simulink model "Regen"  (R2023b)
settings: Solver=VariableStepAuto  StartTime=0.0  StopTime=800.0  RelTol=1e-3
libraries: simulink x1
settings Model: Creator=joser  LastModifiedBy=joser

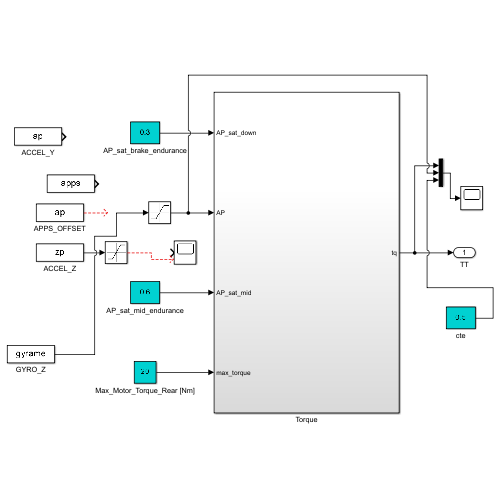
[thumbnail: Simulink's stored preview of the top-level diagram]
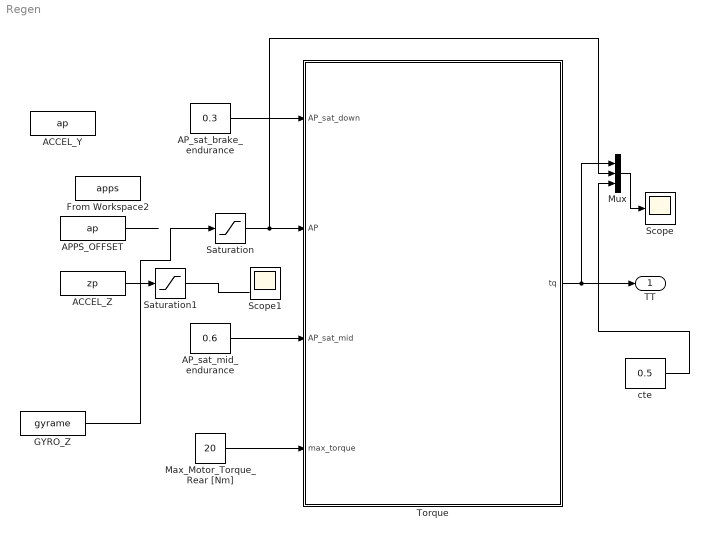
== system Regen ==
  ACCEL_Y : FromWorkspace  VariableName=ap  SampleTime=0.005
  ACCEL_Z : FromWorkspace  VariableName=zp  SampleTime=0.005
  APPS_OFFSET : FromWorkspace  VariableName=ap  SampleTime=0.005
  AP_sat_brake_endurance : Constant  Value=0.3
  AP_sat_mid_endurance : Constant  Value=0.6
  From Workspace2 : FromWorkspace  VariableName=apps  SampleTime=0.005
  GYRO_Z : FromWorkspace  VariableName=gyrame  SampleTime=0.005
  Max_Motor_Torque_Rear [Nm] : Constant  Value=20
  Mux : Mux  Inputs=3
  Saturation : Saturate  UpperLimit=1  LowerLimit=0
  Saturation1 : Saturate  UpperLimit=1  LowerLimit=0
  Scope : Scope
  Scope1 : Scope
  Torque : Subsystem
  cte : Constant  Value=0.5
  TT : Outport
  wires:
  Torque/1(tq) -> Mux/1, TT/1
  AP_sat_brake_endurance/1 -> Torque/1(AP_sat_down)
  Max_Motor_Torque_Rear [Nm]/1 -> Torque/4(max_torque)
  APPS_OFFSET/1 -> ?
  AP_sat_mid_endurance/1 -> Torque/3(AP_sat_mid)
  ACCEL_Z/1 -> Saturation1/1
  Saturation1/1 -> ?
  Mux/1 -> Scope/1
  Saturation/1 -> Mux/2, Torque/2(AP)
  cte/1 -> Mux/3
  GYRO_Z/1 -> Saturation/1

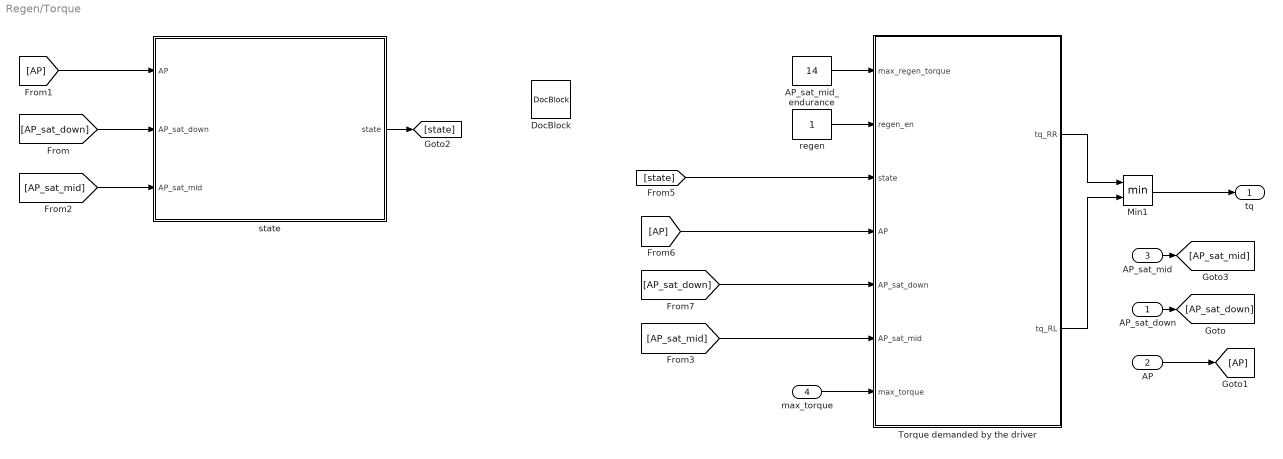
== system Regen/Torque ==
  AP_sat_down : Inport
  AP : Inport  Port=2
  AP_sat_mid : Inport  Port=3
  max_torque : Inport  Port=4
  AP_sat_mid_endurance : Constant  Value=14
  DocBlock : simulink/Model-Wide Utilities/DocBlock  DocumentType=Text
      content=|
      | FUNCIONAMENT DEL SUBSISTEMA
      | per especificacions d'accu, hem de implementar un "lift and coast" per a maximitzar la duració
      | de l'accu i intentar completar la endurance.
      | Per a fer això, s'ha decidit dividir el pedal en 3 zones. Parlarem del recorregut de 0 a 1,
      | sent 0=0º i 1=30º: de 0 a 0.4 el cotxe farà regenerativa, de 0.4 a 0.5 el motor no aplicarà cap força
      | i de 0.5 a 1 el motor accelera el monoplaça.
      |
      | El bloc state determina a quin punt del recorregut del accelerador estem.
      | El bloc regen calcula el torque màxim de frenada que podem aplicar.
      | El bloc torque calcula el torque a aplicar segons l'estat del pedal i els torques de regen.
  Min1 : MinMax  Inputs=2
  Torque demanded by the driver : MATLAB Function  TreatAsAtomicUnit=on
  regen : Constant
  state : MATLAB Function  TreatAsAtomicUnit=on
  tq : Outport
  wires:
  AP_sat_down/1 -> [AP_sat_down]
  [AP_sat_down] -> state/2(AP_sat_down)
  AP/1 -> [AP]
  [AP] -> state/1(AP)
  [AP] -> Torque demanded by the driver/4(AP)
  [AP_sat_down] -> Torque demanded by the driver/5(AP_sat_down)
  state/1(state) -> [state]
  AP_sat_mid_endurance/1 -> Torque demanded by the driver/1(max_regen_torque)
  AP_sat_mid/1 -> [AP_sat_mid]
  [AP_sat_mid] -> state/3(AP_sat_mid)
  [AP_sat_mid] -> Torque demanded by the driver/6(AP_sat_mid)
  Torque demanded by the driver/1(tq_RR) -> Min1/1
  Torque demanded by the driver/2(tq_RL) -> Min1/2
  Min1/1 -> tq/1
  [state] -> Torque demanded by the driver/3(state)
  max_torque/1 -> Torque demanded by the driver/7(max_torque)
  regen/1 -> Torque demanded by the driver/2(regen_en)

== matlab function Regen/Torque/state ==
  data: AP input; AP_sat_down input; state output; AP_sat_mid input
function state = Pedal_State(AP, AP_sat_down, AP_sat_mid)
% state = 0 -> braking
% state = 1 -> lift
% state = 2 -> accelerating
state = 1;
if AP < AP_sat_down
    state = 0;
    return;
end
if AP >= AP_sat_down && AP <= AP_sat_mid
    state = 1;
    return;
end
if AP > AP_sat_mid
    state = 2;
    return;
end
end

== matlab function Regen/Torque/Torque demanded by the driver ==
  data: max_regen_torque input; regen_en input; state input; AP input; AP_sat_down input; AP_sat_mid input; tq_RR output; tq_RL output; max_torque input
function [tq_RR, tq_RL] = torque(max_regen_torque, regen_en, state, AP, AP_sat_down, AP_sat_mid, max_torque)
% state = 0 -> braking
% state = 1 -> lift
% state = 2 -> accelerating
    tq_RR = 0;
    tq_RL = 0;
    if state == 0
        if regen_en == 1
        tq_RR = AP * (max_regen_torque/AP_sat_down) - max_regen_torque;
        tq_RL = tq_RR;
        else
            tq_RR = 0;
            tq_RL = 0;
        end
    end
    if state == 1
        tq_RR = 0;
        tq_RL = 0;
    end
    if state == 2
        tq_RR = max_torque * ((AP-AP_sat_mid) / (1 - AP_sat_mid));
        tq_RL = tq_RR;
    end
end
